simulink model "can8auto"  (R2018a)
settings: Solver=VariableStepAuto  StartTime=0.0  StopTime=5000  RelTol=1e-3
libraries: commcrc2 x20, simulink x20, simulink_extras x5, dspswit3 x5
(part 3 of 7)

== system can8auto/PDO NODO CAN /CAN NODE/NMT Frame generator/11-bit Adder ==
  In1 : Inport
  In2 : Inport  Port=2
  11-bit Adder : Subsystem
  Data Type Conversion : DataTypeConversion
  Demux : Demux  Outputs=11
  Demux1 : Demux  Outputs=11
  Mux : Mux  Inputs=11
  Out1 : Outport
  wires:
  Data Type Conversion/1 -> Out1/1
  Demux1/11 -> 11-bit Adder/22(22)
  Demux1/10 -> 11-bit Adder/21(21)
  Demux1/9 -> 11-bit Adder/20(20)
  Demux1/8 -> 11-bit Adder/19(19)
  Demux1/7 -> 11-bit Adder/18(18)
  Demux1/6 -> 11-bit Adder/17(17)
  Demux1/5 -> 11-bit Adder/16(16)
  Demux1/4 -> 11-bit Adder/15(15)
  Demux1/3 -> 11-bit Adder/14(14)
  Demux1/2 -> 11-bit Adder/13(13)
  Demux1/1 -> 11-bit Adder/12(12)
  Demux/11 -> 11-bit Adder/11(11)
  Demux/10 -> 11-bit Adder/10(10)
  Demux/9 -> 11-bit Adder/9(9)
  Demux/8 -> 11-bit Adder/8(8)
  Demux/7 -> 11-bit Adder/7(7)
  Demux/6 -> 11-bit Adder/6(6)
  Demux/5 -> 11-bit Adder/5(5)
  Demux/4 -> 11-bit Adder/4(4)
  Demux/3 -> 11-bit Adder/3(3)
  Demux/2 -> 11-bit Adder/2(2)
  Demux/1 -> 11-bit Adder/1(1)
  11-bit Adder/11(out11) -> Mux/11
  11-bit Adder/10(out10) -> Mux/10
  11-bit Adder/9(out9) -> Mux/9
  11-bit Adder/8(out8) -> Mux/8
  11-bit Adder/7(out7) -> Mux/7
  11-bit Adder/6(out6) -> Mux/6
  11-bit Adder/5(out5) -> Mux/5
  11-bit Adder/4(out4) -> Mux/4
  11-bit Adder/3(out3) -> Mux/3
  11-bit Adder/2(out2) -> Mux/2
  11-bit Adder/1(out1) -> Mux/1
  In2/1 -> Demux1/1
  In1/1 -> Demux/1
  Mux/1 -> Data Type Conversion/1

== system can8auto/PDO NODO CAN /CAN NODE/NMT Frame generator/BitStuffing ==
  In1 : Inport
  MATLAB Function : MATLAB Function  TreatAsAtomicUnit=on
  Out1 : Outport
  wires:
  In1/1 -> MATLAB Function/1(u)
  MATLAB Function/1(b) -> Out1/1

== system can8auto/PDO NODO CAN /CAN NODE/PDO Frame Generator/Subsystem ==
  Random Bits : Inport
  Length of Field : Inport  Port=2
  1B : Subsystem  TreatAsAtomicUnit=on
  1B1 : Subsystem  TreatAsAtomicUnit=on
  1B2 : Subsystem  TreatAsAtomicUnit=on
  1B3 : Subsystem  TreatAsAtomicUnit=on
  1B4 : Subsystem  TreatAsAtomicUnit=on
  1B5 : Subsystem  TreatAsAtomicUnit=on
  1B6 : Subsystem  TreatAsAtomicUnit=on
  1B7 : Subsystem  TreatAsAtomicUnit=on
  Demux : Demux  Outputs=8
  Index Vector : MultiPortSwitch  Inputs=8  AllowDiffInputSizes=on
  Switch Case : SwitchCase  CaseConditions={1,2,3,4,5,6,7}
  Generated Field : Outport
  wires:
  Switch Case/8 -> 1B7/Action
  1B/1(Out1) -> Index Vector/2
  Demux/3 -> 1B2/3(In3), 1B6/3(In3), 1B4/3(In3), 1B3/3(In3), 1B7/3(In3), 1B5/3(In3)
  Random Bits/1 -> Demux/1
  Switch Case/3 -> 1B2/Action
  Switch Case/6 -> 1B5/Action
  Demux/2 -> 1B2/2(In2), 1B3/2(In2), 1B4/2(In2), 1B5/2(In2), 1B7/2(In2), 1B6/2(In2), 1B1/2(In2)
  1B2/1(Out1) -> Index Vector/4
  Switch Case/5 -> 1B4/Action
  1B3/1(Out1) -> Index Vector/5
  Demux/1 -> 1B1/1(In1), 1B/1(In1), 1B2/1(In1), 1B3/1(In1), 1B4/1(In1), 1B5/1(In1), 1B6/1(In1), 1B7/1(In1)
  Switch Case/2 -> 1B1/Action
  Switch Case/7 -> 1B6/Action
  Demux/4 -> 1B6/4(In4), 1B3/4(In4), 1B7/4(In4), 1B4/4(In4), 1B5/4(In4)
  1B1/1(Out1) -> Index Vector/3
  1B4/1(Out1) -> Index Vector/6
  Demux/8 -> 1B7/8(In8)
  Demux/7 -> 1B6/7(In7), 1B7/7(In7)
  Length of Field/1 -> Switch Case/1, Index Vector/1
  Switch Case/4 -> 1B3/Action
  Demux/5 -> 1B4/5(In5), 1B7/5(In5), 1B6/5(In5), 1B5/5(In5)
  Demux/6 -> 1B5/6(In6), 1B6/6(In6), 1B7/6(In6)
  1B6/1(Out1) -> Index Vector/8
  Switch Case/1 -> 1B/Action
  1B7/1(Out1) -> Index Vector/9
  1B5/1(Out1) -> Index Vector/7
  Index Vector/1 -> Generated Field/1

== system can8auto/PDO NODO CAN /CAN NODE/PDO Frame Generator/Switch Case Action Subsystem ==
  In1 : Inport
  Action Port : ActionPort  ActionType=case
  Out1 : Outport
  wires:
  In1/1 -> Out1/1

== system can8auto/PDO NODO CAN /CAN NODE/PDO Frame Generator/Switch Case Action Subsystem1 ==
  In1 : Inport
  Action Port : ActionPort  ActionType=case
  Out1 : Outport
  wires:
  In1/1 -> Out1/1

== system can8auto/PDO NODO CAN /CAN NODE/PDO Frame Generator/Switch Case Action Subsystem2 ==
  In1 : Inport
  Action Port : ActionPort  ActionType=default
  Out1 : Outport
  wires:
  In1/1 -> Out1/1

== system can8auto/PDO NODO CAN /CAN NODE/SDO Frame generator/BitStuffing ==
  In1 : Inport
  MATLAB Function : MATLAB Function  TreatAsAtomicUnit=on
  Out1 : Outport
  wires:
  In1/1 -> MATLAB Function/1(u)
  MATLAB Function/1(b) -> Out1/1

== system can8auto/PDO NODO CAN /CAN NODE/SDO Frame generator/MUX ==
  Mode : Inport
  Read Client Data : Inport  Port=2
  Write Client Data : Inport  Port=3
  Read Server Data : Inport  Port=4
  Write Server Data : Inport  Port=5
  Complex to Real-Imag : ComplexToRealImag  Output=Real
  MATLAB Function : MATLAB Function  TreatAsAtomicUnit=on
  Vector Concatenate5 : Concatenate  NumInputs=4
  Data to Frame : Outport
  wires:
  Read Server Data/1 -> Vector Concatenate5/3
  Complex to Real-Imag/1 -> Data to Frame/1
  MATLAB Function/1(result) -> Complex to Real-Imag/1
  Read Client Data/1 -> Vector Concatenate5/1
  Vector Concatenate5/1 -> MATLAB Function/2(u1)
  Write Server Data/1 -> Vector Concatenate5/4
  Mode/1 -> MATLAB Function/1(index)
  Write Client Data/1 -> Vector Concatenate5/2

== system can8auto/PDO NODO CAN /CAN NODE/SDO Frame generator/Subsystem ==
  Random Bits : Inport
  Length of Field : Inport  Port=2
  1B : Subsystem  TreatAsAtomicUnit=on
  1B1 : Subsystem  TreatAsAtomicUnit=on
  1B2 : Subsystem  TreatAsAtomicUnit=on
  1B3 : Subsystem  TreatAsAtomicUnit=on
  1B4 : Subsystem  TreatAsAtomicUnit=on
  1B5 : Subsystem  TreatAsAtomicUnit=on
  1B6 : Subsystem  TreatAsAtomicUnit=on
  1B7 : Subsystem  TreatAsAtomicUnit=on
  Demux : Demux  Outputs=8
  Index Vector : MultiPortSwitch  Inputs=8  AllowDiffInputSizes=on
  Switch Case : SwitchCase  CaseConditions={1,2,3,4,5,6,7}
  Generated Field : Outport
  wires:
  Switch Case/8 -> 1B7/Action
  1B/1(Out1) -> Index Vector/2
  Demux/3 -> 1B2/3(In3), 1B6/3(In3), 1B4/3(In3), 1B3/3(In3), 1B7/3(In3), 1B5/3(In3)
  Random Bits/1 -> Demux/1
  Switch Case/3 -> 1B2/Action
  Switch Case/6 -> 1B5/Action
  Demux/2 -> 1B2/2(In2), 1B3/2(In2), 1B4/2(In2), 1B5/2(In2), 1B7/2(In2), 1B6/2(In2), 1B1/2(In2)
  1B2/1(Out1) -> Index Vector/4
  Switch Case/5 -> 1B4/Action
  1B3/1(Out1) -> Index Vector/5
  Demux/1 -> 1B1/1(In1), 1B/1(In1), 1B2/1(In1), 1B3/1(In1), 1B4/1(In1), 1B5/1(In1), 1B6/1(In1), 1B7/1(In1)
  Switch Case/2 -> 1B1/Action
  Switch Case/7 -> 1B6/Action
  Demux/4 -> 1B6/4(In4), 1B3/4(In4), 1B7/4(In4), 1B4/4(In4), 1B5/4(In4)
  1B1/1(Out1) -> Index Vector/3
  1B4/1(Out1) -> Index Vector/6
  Demux/8 -> 1B7/8(In8)
  Demux/7 -> 1B6/7(In7), 1B7/7(In7)
  Length of Field/1 -> Switch Case/1, Index Vector/1
  Switch Case/4 -> 1B3/Action
  Demux/5 -> 1B4/5(In5), 1B7/5(In5), 1B6/5(In5), 1B5/5(In5)
  Demux/6 -> 1B5/6(In6), 1B6/6(In6), 1B7/6(In6)
  1B6/1(Out1) -> Index Vector/8
  Switch Case/1 -> 1B/Action
  1B7/1(Out1) -> Index Vector/9
  1B5/1(Out1) -> Index Vector/7
  Index Vector/1 -> Generated Field/1

== system can8auto/PDO NODO CAN /CAN NODE/SDO Frame generator/Subsystem1 ==
  Random Bits : Inport
  Length of Field : Inport  Port=2
  1B : Subsystem  TreatAsAtomicUnit=on
  1B1 : Subsystem  TreatAsAtomicUnit=on
  1B2 : Subsystem  TreatAsAtomicUnit=on
  1B3 : Subsystem  TreatAsAtomicUnit=on
  1B4 : Subsystem  TreatAsAtomicUnit=on
  1B5 : Subsystem  TreatAsAtomicUnit=on
  1B6 : Subsystem  TreatAsAtomicUnit=on
  1B7 : Subsystem  TreatAsAtomicUnit=on
  Demux : Demux  Outputs=8
  Index Vector : MultiPortSwitch  Inputs=8  AllowDiffInputSizes=on
  Switch Case : SwitchCase  CaseConditions={1,2,3,4,5,6,7}
  Generated Field : Outport
  wires:
  Switch Case/8 -> 1B7/Action
  1B/1(Out1) -> Index Vector/2
  Demux/3 -> 1B2/3(In3), 1B6/3(In3), 1B4/3(In3), 1B3/3(In3), 1B7/3(In3), 1B5/3(In3)
  Random Bits/1 -> Demux/1
  Switch Case/3 -> 1B2/Action
  Switch Case/6 -> 1B5/Action
  Demux/2 -> 1B2/2(In2), 1B3/2(In2), 1B4/2(In2), 1B5/2(In2), 1B7/2(In2), 1B6/2(In2), 1B1/2(In2)
  1B2/1(Out1) -> Index Vector/4
  Switch Case/5 -> 1B4/Action
  1B3/1(Out1) -> Index Vector/5
  Demux/1 -> 1B1/1(In1), 1B/1(In1), 1B2/1(In1), 1B3/1(In1), 1B4/1(In1), 1B5/1(In1), 1B6/1(In1), 1B7/1(In1)
  Switch Case/2 -> 1B1/Action
  Switch Case/7 -> 1B6/Action
  Demux/4 -> 1B6/4(In4), 1B3/4(In4), 1B7/4(In4), 1B4/4(In4), 1B5/4(In4)
  1B1/1(Out1) -> Index Vector/3
  1B4/1(Out1) -> Index Vector/6
  Demux/8 -> 1B7/8(In8)
  Demux/7 -> 1B6/7(In7), 1B7/7(In7)
  Length of Field/1 -> Index Vector/1, Switch Case/1
  Switch Case/4 -> 1B3/Action
  Demux/5 -> 1B4/5(In5), 1B7/5(In5), 1B6/5(In5), 1B5/5(In5)
  Demux/6 -> 1B5/6(In6), 1B6/6(In6), 1B7/6(In6)
  1B6/1(Out1) -> Index Vector/8
  Switch Case/1 -> 1B/Action
  1B7/1(Out1) -> Index Vector/9
  1B5/1(Out1) -> Index Vector/7
  Index Vector/1 -> Generated Field/1

== system can8auto/PDO NODO CAN /CAN NODE/SDO Frame generator/Subsystem2 ==
  Random Bits : Inport
  Length of Field : Inport  Port=2
  1B : Subsystem  TreatAsAtomicUnit=on
  1B1 : Subsystem  TreatAsAtomicUnit=on
  1B2 : Subsystem  TreatAsAtomicUnit=on
  1B3 : Subsystem  TreatAsAtomicUnit=on
  1B4 : Subsystem  TreatAsAtomicUnit=on
  1B5 : Subsystem  TreatAsAtomicUnit=on
  1B6 : Subsystem  TreatAsAtomicUnit=on
  1B7 : Subsystem  TreatAsAtomicUnit=on
  Demux : Demux  Outputs=8
  Index Vector : MultiPortSwitch  Inputs=8  AllowDiffInputSizes=on
  Switch Case : SwitchCase  CaseConditions={1,2,3,4,5,6,7}
  Generated Field : Outport
  wires:
  Switch Case/8 -> 1B7/Action
  1B/1(Out1) -> Index Vector/2
  Demux/3 -> 1B2/3(In3), 1B6/3(In3), 1B4/3(In3), 1B3/3(In3), 1B7/3(In3), 1B5/3(In3)
  Random Bits/1 -> Demux/1
  Switch Case/3 -> 1B2/Action
  Switch Case/6 -> 1B5/Action
  Demux/2 -> 1B2/2(In2), 1B3/2(In2), 1B4/2(In2), 1B5/2(In2), 1B7/2(In2), 1B6/2(In2), 1B1/2(In2)
  1B2/1(Out1) -> Index Vector/4
  Switch Case/5 -> 1B4/Action
  1B3/1(Out1) -> Index Vector/5
  Demux/1 -> 1B1/1(In1), 1B/1(In1), 1B2/1(In1), 1B3/1(In1), 1B4/1(In1), 1B5/1(In1), 1B6/1(In1), 1B7/1(In1)
  Switch Case/2 -> 1B1/Action
  Switch Case/7 -> 1B6/Action
  Demux/4 -> 1B6/4(In4), 1B3/4(In4), 1B7/4(In4), 1B4/4(In4), 1B5/4(In4)
  1B1/1(Out1) -> Index Vector/3
  1B4/1(Out1) -> Index Vector/6
  Demux/8 -> 1B7/8(In8)
  Demux/7 -> 1B6/7(In7), 1B7/7(In7)
  Length of Field/1 -> Switch Case/1, Index Vector/1
  Switch Case/4 -> 1B3/Action
  Demux/5 -> 1B4/5(In5), 1B7/5(In5), 1B6/5(In5), 1B5/5(In5)
  Demux/6 -> 1B5/6(In6), 1B6/6(In6), 1B7/6(In6)
  1B6/1(Out1) -> Index Vector/8
  Switch Case/1 -> 1B/Action
  1B7/1(Out1) -> Index Vector/9
  1B5/1(Out1) -> Index Vector/7
  Index Vector/1 -> Generated Field/1

== system can8auto/PDO NODO CAN /CAN NODE/SDO Frame generator/Subsystem3 ==
  Random Bits : Inport
  Length of Field : Inport  Port=2
  1B : Subsystem  TreatAsAtomicUnit=on
  1B1 : Subsystem  TreatAsAtomicUnit=on
  1B2 : Subsystem  TreatAsAtomicUnit=on
  1B3 : Subsystem  TreatAsAtomicUnit=on
  1B4 : Subsystem  TreatAsAtomicUnit=on
  1B5 : Subsystem  TreatAsAtomicUnit=on
  1B6 : Subsystem  TreatAsAtomicUnit=on
  1B7 : Subsystem  TreatAsAtomicUnit=on
  Demux : Demux  Outputs=8
  Index Vector : MultiPortSwitch  Inputs=8  AllowDiffInputSizes=on
  Switch Case : SwitchCase  CaseConditions={1,2,3,4,5,6,7}
  Generated Field : Outport
  wires:
  Switch Case/8 -> 1B7/Action
  1B/1(Out1) -> Index Vector/2
  Demux/3 -> 1B2/3(In3), 1B6/3(In3), 1B4/3(In3), 1B3/3(In3), 1B7/3(In3), 1B5/3(In3)
  Random Bits/1 -> Demux/1
  Switch Case/3 -> 1B2/Action
  Switch Case/6 -> 1B5/Action
  Demux/2 -> 1B2/2(In2), 1B3/2(In2), 1B4/2(In2), 1B5/2(In2), 1B7/2(In2), 1B6/2(In2), 1B1/2(In2)
  1B2/1(Out1) -> Index Vector/4
  Switch Case/5 -> 1B4/Action
  1B3/1(Out1) -> Index Vector/5
  Demux/1 -> 1B1/1(In1), 1B/1(In1), 1B2/1(In1), 1B3/1(In1), 1B4/1(In1), 1B5/1(In1), 1B6/1(In1), 1B7/1(In1)
  Switch Case/2 -> 1B1/Action
  Switch Case/7 -> 1B6/Action
  Demux/4 -> 1B6/4(In4), 1B3/4(In4), 1B7/4(In4), 1B4/4(In4), 1B5/4(In4)
  1B1/1(Out1) -> Index Vector/3
  1B4/1(Out1) -> Index Vector/6
  Demux/8 -> 1B7/8(In8)
  Demux/7 -> 1B6/7(In7), 1B7/7(In7)
  Length of Field/1 -> Switch Case/1, Index Vector/1
  Switch Case/4 -> 1B3/Action
  Demux/5 -> 1B4/5(In5), 1B7/5(In5), 1B6/5(In5), 1B5/5(In5)
  Demux/6 -> 1B5/6(In6), 1B6/6(In6), 1B7/6(In6)
  1B6/1(Out1) -> Index Vector/8
  Switch Case/1 -> 1B/Action
  1B7/1(Out1) -> Index Vector/9
  1B5/1(Out1) -> Index Vector/7
  Index Vector/1 -> Generated Field/1

== system can8auto/PDO NODO CAN /CAN NODE/SYNC Frame Generator/BitStuffing ==
  In1 : Inport
  MATLAB Function : MATLAB Function  TreatAsAtomicUnit=on
  Out1 : Outport
  wires:
  In1/1 -> MATLAB Function/1(u)
  MATLAB Function/1(b) -> Out1/1

== system can8auto/SDO NODO CAN/CAN NODE/Bootup Frame generator/11-bit Adder ==
  In1 : Inport
  In2 : Inport  Port=2
  8-bit Adder : Subsystem
  Data Type Conversion : DataTypeConversion
  Demux : Demux  Outputs=11
  Demux1 : Demux  Outputs=11
  Mux : Mux  Inputs=11
  Out1 : Outport
  wires:
  Data Type Conversion/1 -> Out1/1
  Mux/1 -> Data Type Conversion/1
  Demux1/11 -> 8-bit Adder/22(22)
  Demux1/10 -> 8-bit Adder/21(21)
  Demux1/9 -> 8-bit Adder/20(20)
  Demux1/8 -> 8-bit Adder/19(19)
  Demux1/7 -> 8-bit Adder/18(18)
  Demux1/6 -> 8-bit Adder/17(17)
  Demux1/5 -> 8-bit Adder/16(16)
  Demux1/4 -> 8-bit Adder/15(15)
  Demux1/3 -> 8-bit Adder/14(14)
  Demux1/2 -> 8-bit Adder/13(13)
  Demux1/1 -> 8-bit Adder/12(12)
  Demux/11 -> 8-bit Adder/11(11)
  Demux/10 -> 8-bit Adder/10(10)
  Demux/9 -> 8-bit Adder/9(9)
  Demux/8 -> 8-bit Adder/8(8)
  Demux/7 -> 8-bit Adder/7(7)
  Demux/6 -> 8-bit Adder/6(6)
  Demux/5 -> 8-bit Adder/5(5)
  Demux/4 -> 8-bit Adder/4(4)
  Demux/3 -> 8-bit Adder/3(3)
  Demux/2 -> 8-bit Adder/2(2)
  Demux/1 -> 8-bit Adder/1(1)
  8-bit Adder/11(out11) -> Mux/11
  8-bit Adder/10(out10) -> Mux/10
  8-bit Adder/9(out9) -> Mux/9
  8-bit Adder/8(out8) -> Mux/8
  8-bit Adder/7(out7) -> Mux/7
  8-bit Adder/6(out6) -> Mux/6
  8-bit Adder/5(out5) -> Mux/5
  8-bit Adder/4(out4) -> Mux/4
  8-bit Adder/3(out3) -> Mux/3
  8-bit Adder/2(out2) -> Mux/2
  8-bit Adder/1(out1) -> Mux/1
  In2/1 -> Demux1/1
  In1/1 -> Demux/1

== system can8auto/SDO NODO CAN/CAN NODE/Bootup Frame generator/BitStuffing ==
  In1 : Inport
  MATLAB Function : MATLAB Function  TreatAsAtomicUnit=on
  Out1 : Outport
  wires:
  In1/1 -> MATLAB Function/1(u)
  MATLAB Function/1(b) -> Out1/1

== system can8auto/SDO NODO CAN/CAN NODE/NMT Frame generator/11-bit Adder ==
  In1 : Inport
  In2 : Inport  Port=2
  11-bit Adder : Subsystem
  Data Type Conversion : DataTypeConversion
  Demux : Demux  Outputs=11
  Demux1 : Demux  Outputs=11
  Mux : Mux  Inputs=11
  Out1 : Outport
  wires:
  Data Type Conversion/1 -> Out1/1
  Demux1/11 -> 11-bit Adder/22(22)
  Demux1/10 -> 11-bit Adder/21(21)
  Demux1/9 -> 11-bit Adder/20(20)
  Demux1/8 -> 11-bit Adder/19(19)
  Demux1/7 -> 11-bit Adder/18(18)
  Demux1/6 -> 11-bit Adder/17(17)
  Demux1/5 -> 11-bit Adder/16(16)
  Demux1/4 -> 11-bit Adder/15(15)
  Demux1/3 -> 11-bit Adder/14(14)
  Demux1/2 -> 11-bit Adder/13(13)
  Demux1/1 -> 11-bit Adder/12(12)
  Demux/11 -> 11-bit Adder/11(11)
  Demux/10 -> 11-bit Adder/10(10)
  Demux/9 -> 11-bit Adder/9(9)
  Demux/8 -> 11-bit Adder/8(8)
  Demux/7 -> 11-bit Adder/7(7)
  Demux/6 -> 11-bit Adder/6(6)
  Demux/5 -> 11-bit Adder/5(5)
  Demux/4 -> 11-bit Adder/4(4)
  Demux/3 -> 11-bit Adder/3(3)
  Demux/2 -> 11-bit Adder/2(2)
  Demux/1 -> 11-bit Adder/1(1)
  11-bit Adder/11(out11) -> Mux/11
  11-bit Adder/10(out10) -> Mux/10
  11-bit Adder/9(out9) -> Mux/9
  11-bit Adder/8(out8) -> Mux/8
  11-bit Adder/7(out7) -> Mux/7
  11-bit Adder/6(out6) -> Mux/6
  11-bit Adder/5(out5) -> Mux/5
  11-bit Adder/4(out4) -> Mux/4
  11-bit Adder/3(out3) -> Mux/3
  11-bit Adder/2(out2) -> Mux/2
  11-bit Adder/1(out1) -> Mux/1
  In2/1 -> Demux1/1
  In1/1 -> Demux/1
  Mux/1 -> Data Type Conversion/1

== system can8auto/SDO NODO CAN/CAN NODE/NMT Frame generator/BitStuffing ==
  In1 : Inport
  MATLAB Function : MATLAB Function  TreatAsAtomicUnit=on
  Out1 : Outport
  wires:
  In1/1 -> MATLAB Function/1(u)
  MATLAB Function/1(b) -> Out1/1

== system can8auto/SDO NODO CAN/CAN NODE/PDO Frame Generator/Subsystem ==
  Random Bits : Inport
  Length of Field : Inport  Port=2
  1B : Subsystem  TreatAsAtomicUnit=on
  1B1 : Subsystem  TreatAsAtomicUnit=on
  1B2 : Subsystem  TreatAsAtomicUnit=on
  1B3 : Subsystem  TreatAsAtomicUnit=on
  1B4 : Subsystem  TreatAsAtomicUnit=on
  1B5 : Subsystem  TreatAsAtomicUnit=on
  1B6 : Subsystem  TreatAsAtomicUnit=on
  1B7 : Subsystem  TreatAsAtomicUnit=on
  Demux : Demux  Outputs=8
  Index Vector : MultiPortSwitch  Inputs=8  AllowDiffInputSizes=on
  Switch Case : SwitchCase  CaseConditions={1,2,3,4,5,6,7}
  Generated Field : Outport
  wires:
  Switch Case/8 -> 1B7/Action
  1B/1(Out1) -> Index Vector/2
  Demux/3 -> 1B2/3(In3), 1B6/3(In3), 1B4/3(In3), 1B3/3(In3), 1B7/3(In3), 1B5/3(In3)
  Random Bits/1 -> Demux/1
  Switch Case/3 -> 1B2/Action
  Switch Case/6 -> 1B5/Action
  Demux/2 -> 1B2/2(In2), 1B3/2(In2), 1B4/2(In2), 1B5/2(In2), 1B7/2(In2), 1B6/2(In2), 1B1/2(In2)
  1B2/1(Out1) -> Index Vector/4
  Switch Case/5 -> 1B4/Action
  1B3/1(Out1) -> Index Vector/5
  Demux/1 -> 1B1/1(In1), 1B/1(In1), 1B2/1(In1), 1B3/1(In1), 1B4/1(In1), 1B5/1(In1), 1B6/1(In1), 1B7/1(In1)
  Switch Case/2 -> 1B1/Action
  Switch Case/7 -> 1B6/Action
  Demux/4 -> 1B6/4(In4), 1B3/4(In4), 1B7/4(In4), 1B4/4(In4), 1B5/4(In4)
  1B1/1(Out1) -> Index Vector/3
  1B4/1(Out1) -> Index Vector/6
  Demux/8 -> 1B7/8(In8)
  Demux/7 -> 1B6/7(In7), 1B7/7(In7)
  Length of Field/1 -> Switch Case/1, Index Vector/1
  Switch Case/4 -> 1B3/Action
  Demux/5 -> 1B4/5(In5), 1B7/5(In5), 1B6/5(In5), 1B5/5(In5)
  Demux/6 -> 1B5/6(In6), 1B6/6(In6), 1B7/6(In6)
  1B6/1(Out1) -> Index Vector/8
  Switch Case/1 -> 1B/Action
  1B7/1(Out1) -> Index Vector/9
  1B5/1(Out1) -> Index Vector/7
  Index Vector/1 -> Generated Field/1

== system can8auto/SDO NODO CAN/CAN NODE/PDO Frame Generator/Switch Case Action Subsystem ==
  In1 : Inport
  Action Port : ActionPort  ActionType=case
  Out1 : Outport
  wires:
  In1/1 -> Out1/1

== system can8auto/SDO NODO CAN/CAN NODE/PDO Frame Generator/Switch Case Action Subsystem1 ==
  In1 : Inport
  Action Port : ActionPort  ActionType=case
  Out1 : Outport
  wires:
  In1/1 -> Out1/1

== system can8auto/SDO NODO CAN/CAN NODE/PDO Frame Generator/Switch Case Action Subsystem2 ==
  In1 : Inport
  Action Port : ActionPort  ActionType=default
  Out1 : Outport
  wires:
  In1/1 -> Out1/1

== system can8auto/SDO NODO CAN/CAN NODE/SDO Frame generator/BitStuffing ==
  In1 : Inport
  MATLAB Function : MATLAB Function  TreatAsAtomicUnit=on
  Out1 : Outport
  wires:
  In1/1 -> MATLAB Function/1(u)
  MATLAB Function/1(b) -> Out1/1

== system can8auto/SDO NODO CAN/CAN NODE/SDO Frame generator/MUX ==
  Mode : Inport
  Read Client Data : Inport  Port=2
  Write Client Data : Inport  Port=3
  Read Server Data : Inport  Port=4
  Write Server Data : Inport  Port=5
  Complex to Real-Imag : ComplexToRealImag  Output=Real
  MATLAB Function : MATLAB Function  TreatAsAtomicUnit=on
  Vector Concatenate5 : Concatenate  NumInputs=4
  Data to Frame : Outport
  wires:
  Read Server Data/1 -> Vector Concatenate5/3
  Complex to Real-Imag/1 -> Data to Frame/1
  MATLAB Function/1(result) -> Complex to Real-Imag/1
  Read Client Data/1 -> Vector Concatenate5/1
  Vector Concatenate5/1 -> MATLAB Function/2(u1)
  Write Server Data/1 -> Vector Concatenate5/4
  Mode/1 -> MATLAB Function/1(index)
  Write Client Data/1 -> Vector Concatenate5/2

== system can8auto/SDO NODO CAN/CAN NODE/SDO Frame generator/Subsystem ==
  Random Bits : Inport
  Length of Field : Inport  Port=2
  1B : Subsystem  TreatAsAtomicUnit=on
  1B1 : Subsystem  TreatAsAtomicUnit=on
  1B2 : Subsystem  TreatAsAtomicUnit=on
  1B3 : Subsystem  TreatAsAtomicUnit=on
  1B4 : Subsystem  TreatAsAtomicUnit=on
  1B5 : Subsystem  TreatAsAtomicUnit=on
  1B6 : Subsystem  TreatAsAtomicUnit=on
  1B7 : Subsystem  TreatAsAtomicUnit=on
  Demux : Demux  Outputs=8
  Index Vector : MultiPortSwitch  Inputs=8  AllowDiffInputSizes=on
  Switch Case : SwitchCase  CaseConditions={1,2,3,4,5,6,7}
  Generated Field : Outport
  wires:
  Switch Case/8 -> 1B7/Action
  1B/1(Out1) -> Index Vector/2
  Demux/3 -> 1B2/3(In3), 1B6/3(In3), 1B4/3(In3), 1B3/3(In3), 1B7/3(In3), 1B5/3(In3)
  Random Bits/1 -> Demux/1
  Switch Case/3 -> 1B2/Action
  Switch Case/6 -> 1B5/Action
  Demux/2 -> 1B2/2(In2), 1B3/2(In2), 1B4/2(In2), 1B5/2(In2), 1B7/2(In2), 1B6/2(In2), 1B1/2(In2)
  1B2/1(Out1) -> Index Vector/4
  Switch Case/5 -> 1B4/Action
  1B3/1(Out1) -> Index Vector/5
  Demux/1 -> 1B1/1(In1), 1B/1(In1), 1B2/1(In1), 1B3/1(In1), 1B4/1(In1), 1B5/1(In1), 1B6/1(In1), 1B7/1(In1)
  Switch Case/2 -> 1B1/Action
  Switch Case/7 -> 1B6/Action
  Demux/4 -> 1B6/4(In4), 1B3/4(In4), 1B7/4(In4), 1B4/4(In4), 1B5/4(In4)
  1B1/1(Out1) -> Index Vector/3
  1B4/1(Out1) -> Index Vector/6
  Demux/8 -> 1B7/8(In8)
  Demux/7 -> 1B6/7(In7), 1B7/7(In7)
  Length of Field/1 -> Switch Case/1, Index Vector/1
  Switch Case/4 -> 1B3/Action
  Demux/5 -> 1B4/5(In5), 1B7/5(In5), 1B6/5(In5), 1B5/5(In5)
  Demux/6 -> 1B5/6(In6), 1B6/6(In6), 1B7/6(In6)
  1B6/1(Out1) -> Index Vector/8
  Switch Case/1 -> 1B/Action
  1B7/1(Out1) -> Index Vector/9
  1B5/1(Out1) -> Index Vector/7
  Index Vector/1 -> Generated Field/1

== system can8auto/SDO NODO CAN/CAN NODE/SDO Frame generator/Subsystem1 ==
  Random Bits : Inport
  Length of Field : Inport  Port=2
  1B : Subsystem  TreatAsAtomicUnit=on
  1B1 : Subsystem  TreatAsAtomicUnit=on
  1B2 : Subsystem  TreatAsAtomicUnit=on
  1B3 : Subsystem  TreatAsAtomicUnit=on
  1B4 : Subsystem  TreatAsAtomicUnit=on
  1B5 : Subsystem  TreatAsAtomicUnit=on
  1B6 : Subsystem  TreatAsAtomicUnit=on
  1B7 : Subsystem  TreatAsAtomicUnit=on
  Demux : Demux  Outputs=8
  Index Vector : MultiPortSwitch  Inputs=8  AllowDiffInputSizes=on
  Switch Case : SwitchCase  CaseConditions={1,2,3,4,5,6,7}
  Generated Field : Outport
  wires:
  Switch Case/8 -> 1B7/Action
  1B/1(Out1) -> Index Vector/2
  Demux/3 -> 1B2/3(In3), 1B6/3(In3), 1B4/3(In3), 1B3/3(In3), 1B7/3(In3), 1B5/3(In3)
  Random Bits/1 -> Demux/1
  Switch Case/3 -> 1B2/Action
  Switch Case/6 -> 1B5/Action
  Demux/2 -> 1B2/2(In2), 1B3/2(In2), 1B4/2(In2), 1B5/2(In2), 1B7/2(In2), 1B6/2(In2), 1B1/2(In2)
  1B2/1(Out1) -> Index Vector/4
  Switch Case/5 -> 1B4/Action
  1B3/1(Out1) -> Index Vector/5
  Demux/1 -> 1B1/1(In1), 1B/1(In1), 1B2/1(In1), 1B3/1(In1), 1B4/1(In1), 1B5/1(In1), 1B6/1(In1), 1B7/1(In1)
  Switch Case/2 -> 1B1/Action
  Switch Case/7 -> 1B6/Action
  Demux/4 -> 1B6/4(In4), 1B3/4(In4), 1B7/4(In4), 1B4/4(In4), 1B5/4(In4)
  1B1/1(Out1) -> Index Vector/3
  1B4/1(Out1) -> Index Vector/6
  Demux/8 -> 1B7/8(In8)
  Demux/7 -> 1B6/7(In7), 1B7/7(In7)
  Length of Field/1 -> Index Vector/1, Switch Case/1
  Switch Case/4 -> 1B3/Action
  Demux/5 -> 1B4/5(In5), 1B7/5(In5), 1B6/5(In5), 1B5/5(In5)
  Demux/6 -> 1B5/6(In6), 1B6/6(In6), 1B7/6(In6)
  1B6/1(Out1) -> Index Vector/8
  Switch Case/1 -> 1B/Action
  1B7/1(Out1) -> Index Vector/9
  1B5/1(Out1) -> Index Vector/7
  Index Vector/1 -> Generated Field/1

== system can8auto/SDO NODO CAN/CAN NODE/SDO Frame generator/Subsystem2 ==
  Random Bits : Inport
  Length of Field : Inport  Port=2
  1B : Subsystem  TreatAsAtomicUnit=on
  1B1 : Subsystem  TreatAsAtomicUnit=on
  1B2 : Subsystem  TreatAsAtomicUnit=on
  1B3 : Subsystem  TreatAsAtomicUnit=on
  1B4 : Subsystem  TreatAsAtomicUnit=on
  1B5 : Subsystem  TreatAsAtomicUnit=on
  1B6 : Subsystem  TreatAsAtomicUnit=on
  1B7 : Subsystem  TreatAsAtomicUnit=on
  Demux : Demux  Outputs=8
  Index Vector : MultiPortSwitch  Inputs=8  AllowDiffInputSizes=on
  Switch Case : SwitchCase  CaseConditions={1,2,3,4,5,6,7}
  Generated Field : Outport
  wires:
  Switch Case/8 -> 1B7/Action
  1B/1(Out1) -> Index Vector/2
  Demux/3 -> 1B2/3(In3), 1B6/3(In3), 1B4/3(In3), 1B3/3(In3), 1B7/3(In3), 1B5/3(In3)
  Random Bits/1 -> Demux/1
  Switch Case/3 -> 1B2/Action
  Switch Case/6 -> 1B5/Action
  Demux/2 -> 1B2/2(In2), 1B3/2(In2), 1B4/2(In2), 1B5/2(In2), 1B7/2(In2), 1B6/2(In2), 1B1/2(In2)
  1B2/1(Out1) -> Index Vector/4
  Switch Case/5 -> 1B4/Action
  1B3/1(Out1) -> Index Vector/5
  Demux/1 -> 1B1/1(In1), 1B/1(In1), 1B2/1(In1), 1B3/1(In1), 1B4/1(In1), 1B5/1(In1), 1B6/1(In1), 1B7/1(In1)
  Switch Case/2 -> 1B1/Action
  Switch Case/7 -> 1B6/Action
  Demux/4 -> 1B6/4(In4), 1B3/4(In4), 1B7/4(In4), 1B4/4(In4), 1B5/4(In4)
  1B1/1(Out1) -> Index Vector/3
  1B4/1(Out1) -> Index Vector/6
  Demux/8 -> 1B7/8(In8)
  Demux/7 -> 1B6/7(In7), 1B7/7(In7)
  Length of Field/1 -> Switch Case/1, Index Vector/1
  Switch Case/4 -> 1B3/Action
  Demux/5 -> 1B4/5(In5), 1B7/5(In5), 1B6/5(In5), 1B5/5(In5)
  Demux/6 -> 1B5/6(In6), 1B6/6(In6), 1B7/6(In6)
  1B6/1(Out1) -> Index Vector/8
  Switch Case/1 -> 1B/Action
  1B7/1(Out1) -> Index Vector/9
  1B5/1(Out1) -> Index Vector/7
  Index Vector/1 -> Generated Field/1

== system can8auto/SDO NODO CAN/CAN NODE/SDO Frame generator/Subsystem3 ==
  Random Bits : Inport
  Length of Field : Inport  Port=2
  1B : Subsystem  TreatAsAtomicUnit=on
  1B1 : Subsystem  TreatAsAtomicUnit=on
  1B2 : Subsystem  TreatAsAtomicUnit=on
  1B3 : Subsystem  TreatAsAtomicUnit=on
  1B4 : Subsystem  TreatAsAtomicUnit=on
  1B5 : Subsystem  TreatAsAtomicUnit=on
  1B6 : Subsystem  TreatAsAtomicUnit=on
  1B7 : Subsystem  TreatAsAtomicUnit=on
  Demux : Demux  Outputs=8
  Index Vector : MultiPortSwitch  Inputs=8  AllowDiffInputSizes=on
  Switch Case : SwitchCase  CaseConditions={1,2,3,4,5,6,7}
  Generated Field : Outport
  wires:
  Switch Case/8 -> 1B7/Action
  1B/1(Out1) -> Index Vector/2
  Demux/3 -> 1B2/3(In3), 1B6/3(In3), 1B4/3(In3), 1B3/3(In3), 1B7/3(In3), 1B5/3(In3)
  Random Bits/1 -> Demux/1
  Switch Case/3 -> 1B2/Action
  Switch Case/6 -> 1B5/Action
  Demux/2 -> 1B2/2(In2), 1B3/2(In2), 1B4/2(In2), 1B5/2(In2), 1B7/2(In2), 1B6/2(In2), 1B1/2(In2)
  1B2/1(Out1) -> Index Vector/4
  Switch Case/5 -> 1B4/Action
  1B3/1(Out1) -> Index Vector/5
  Demux/1 -> 1B1/1(In1), 1B/1(In1), 1B2/1(In1), 1B3/1(In1), 1B4/1(In1), 1B5/1(In1), 1B6/1(In1), 1B7/1(In1)
  Switch Case/2 -> 1B1/Action
  Switch Case/7 -> 1B6/Action
  Demux/4 -> 1B6/4(In4), 1B3/4(In4), 1B7/4(In4), 1B4/4(In4), 1B5/4(In4)
  1B1/1(Out1) -> Index Vector/3
  1B4/1(Out1) -> Index Vector/6
  Demux/8 -> 1B7/8(In8)
  Demux/7 -> 1B6/7(In7), 1B7/7(In7)
  Length of Field/1 -> Switch Case/1, Index Vector/1
  Switch Case/4 -> 1B3/Action
  Demux/5 -> 1B4/5(In5), 1B7/5(In5), 1B6/5(In5), 1B5/5(In5)
  Demux/6 -> 1B5/6(In6), 1B6/6(In6), 1B7/6(In6)
  1B6/1(Out1) -> Index Vector/8
  Switch Case/1 -> 1B/Action
  1B7/1(Out1) -> Index Vector/9
  1B5/1(Out1) -> Index Vector/7
  Index Vector/1 -> Generated Field/1

== system can8auto/SDO NODO CAN/CAN NODE/SYNC Frame Generator/BitStuffing ==
  In1 : Inport
  MATLAB Function : MATLAB Function  TreatAsAtomicUnit=on
  Out1 : Outport
  wires:
  In1/1 -> MATLAB Function/1(u)
  MATLAB Function/1(b) -> Out1/1

== system can8auto/SYNC PRODUCER/CAN NODE/Bootup Frame generator/11-bit Adder ==
  In1 : Inport
  In2 : Inport  Port=2
  8-bit Adder : Subsystem
  Data Type Conversion : DataTypeConversion
  Demux : Demux  Outputs=11
  Demux1 : Demux  Outputs=11
  Mux : Mux  Inputs=11
  Out1 : Outport
  wires:
  Data Type Conversion/1 -> Out1/1
  Mux/1 -> Data Type Conversion/1
  Demux1/11 -> 8-bit Adder/22(22)
  Demux1/10 -> 8-bit Adder/21(21)
  Demux1/9 -> 8-bit Adder/20(20)
  Demux1/8 -> 8-bit Adder/19(19)
  Demux1/7 -> 8-bit Adder/18(18)
  Demux1/6 -> 8-bit Adder/17(17)
  Demux1/5 -> 8-bit Adder/16(16)
  Demux1/4 -> 8-bit Adder/15(15)
  Demux1/3 -> 8-bit Adder/14(14)
  Demux1/2 -> 8-bit Adder/13(13)
  Demux1/1 -> 8-bit Adder/12(12)
  Demux/11 -> 8-bit Adder/11(11)
  Demux/10 -> 8-bit Adder/10(10)
  Demux/9 -> 8-bit Adder/9(9)
  Demux/8 -> 8-bit Adder/8(8)
  Demux/7 -> 8-bit Adder/7(7)
  Demux/6 -> 8-bit Adder/6(6)
  Demux/5 -> 8-bit Adder/5(5)
  Demux/4 -> 8-bit Adder/4(4)
  Demux/3 -> 8-bit Adder/3(3)
  Demux/2 -> 8-bit Adder/2(2)
  Demux/1 -> 8-bit Adder/1(1)
  8-bit Adder/11(out11) -> Mux/11
  8-bit Adder/10(out10) -> Mux/10
  8-bit Adder/9(out9) -> Mux/9
  8-bit Adder/8(out8) -> Mux/8
  8-bit Adder/7(out7) -> Mux/7
  8-bit Adder/6(out6) -> Mux/6
  8-bit Adder/5(out5) -> Mux/5
  8-bit Adder/4(out4) -> Mux/4
  8-bit Adder/3(out3) -> Mux/3
  8-bit Adder/2(out2) -> Mux/2
  8-bit Adder/1(out1) -> Mux/1
  In2/1 -> Demux1/1
  In1/1 -> Demux/1

== system can8auto/SYNC PRODUCER/CAN NODE/Bootup Frame generator/BitStuffing ==
  In1 : Inport
  MATLAB Function : MATLAB Function  TreatAsAtomicUnit=on
  Out1 : Outport
  wires:
  In1/1 -> MATLAB Function/1(u)
  MATLAB Function/1(b) -> Out1/1

== system can8auto/SYNC PRODUCER/CAN NODE/NMT Frame generator/11-bit Adder ==
  In1 : Inport
  In2 : Inport  Port=2
  11-bit Adder : Subsystem
  Data Type Conversion : DataTypeConversion
  Demux : Demux  Outputs=11
  Demux1 : Demux  Outputs=11
  Mux : Mux  Inputs=11
  Out1 : Outport
  wires:
  Data Type Conversion/1 -> Out1/1
  Demux1/11 -> 11-bit Adder/22(22)
  Demux1/10 -> 11-bit Adder/21(21)
  Demux1/9 -> 11-bit Adder/20(20)
  Demux1/8 -> 11-bit Adder/19(19)
  Demux1/7 -> 11-bit Adder/18(18)
  Demux1/6 -> 11-bit Adder/17(17)
  Demux1/5 -> 11-bit Adder/16(16)
  Demux1/4 -> 11-bit Adder/15(15)
  Demux1/3 -> 11-bit Adder/14(14)
  Demux1/2 -> 11-bit Adder/13(13)
  Demux1/1 -> 11-bit Adder/12(12)
  Demux/11 -> 11-bit Adder/11(11)
  Demux/10 -> 11-bit Adder/10(10)
  Demux/9 -> 11-bit Adder/9(9)
  Demux/8 -> 11-bit Adder/8(8)
  Demux/7 -> 11-bit Adder/7(7)
  Demux/6 -> 11-bit Adder/6(6)
  Demux/5 -> 11-bit Adder/5(5)
  Demux/4 -> 11-bit Adder/4(4)
  Demux/3 -> 11-bit Adder/3(3)
  Demux/2 -> 11-bit Adder/2(2)
  Demux/1 -> 11-bit Adder/1(1)
  11-bit Adder/11(out11) -> Mux/11
  11-bit Adder/10(out10) -> Mux/10
  11-bit Adder/9(out9) -> Mux/9
  11-bit Adder/8(out8) -> Mux/8
  11-bit Adder/7(out7) -> Mux/7
  11-bit Adder/6(out6) -> Mux/6
  11-bit Adder/5(out5) -> Mux/5
  11-bit Adder/4(out4) -> Mux/4
  11-bit Adder/3(out3) -> Mux/3
  11-bit Adder/2(out2) -> Mux/2
  11-bit Adder/1(out1) -> Mux/1
  In2/1 -> Demux1/1
  In1/1 -> Demux/1
  Mux/1 -> Data Type Conversion/1

== system can8auto/SYNC PRODUCER/CAN NODE/NMT Frame generator/BitStuffing ==
  In1 : Inport
  MATLAB Function : MATLAB Function  TreatAsAtomicUnit=on
  Out1 : Outport
  wires:
  In1/1 -> MATLAB Function/1(u)
  MATLAB Function/1(b) -> Out1/1

== system can8auto/SYNC PRODUCER/CAN NODE/PDO Frame Generator/Subsystem ==
  Random Bits : Inport
  Length of Field : Inport  Port=2
  1B : Subsystem  TreatAsAtomicUnit=on
  1B1 : Subsystem  TreatAsAtomicUnit=on
  1B2 : Subsystem  TreatAsAtomicUnit=on
  1B3 : Subsystem  TreatAsAtomicUnit=on
  1B4 : Subsystem  TreatAsAtomicUnit=on
  1B5 : Subsystem  TreatAsAtomicUnit=on
  1B6 : Subsystem  TreatAsAtomicUnit=on
  1B7 : Subsystem  TreatAsAtomicUnit=on
  Demux : Demux  Outputs=8
  Index Vector : MultiPortSwitch  Inputs=8  AllowDiffInputSizes=on
  Switch Case : SwitchCase  CaseConditions={1,2,3,4,5,6,7}
  Generated Field : Outport
  wires:
  Switch Case/8 -> 1B7/Action
  1B/1(Out1) -> Index Vector/2
  Demux/3 -> 1B2/3(In3), 1B6/3(In3), 1B4/3(In3), 1B3/3(In3), 1B7/3(In3), 1B5/3(In3)
  Random Bits/1 -> Demux/1
  Switch Case/3 -> 1B2/Action
  Switch Case/6 -> 1B5/Action
  Demux/2 -> 1B2/2(In2), 1B3/2(In2), 1B4/2(In2), 1B5/2(In2), 1B7/2(In2), 1B6/2(In2), 1B1/2(In2)
  1B2/1(Out1) -> Index Vector/4
  Switch Case/5 -> 1B4/Action
  1B3/1(Out1) -> Index Vector/5
  Demux/1 -> 1B1/1(In1), 1B/1(In1), 1B2/1(In1), 1B3/1(In1), 1B4/1(In1), 1B5/1(In1), 1B6/1(In1), 1B7/1(In1)
  Switch Case/2 -> 1B1/Action
  Switch Case/7 -> 1B6/Action
  Demux/4 -> 1B6/4(In4), 1B3/4(In4), 1B7/4(In4), 1B4/4(In4), 1B5/4(In4)
  1B1/1(Out1) -> Index Vector/3
  1B4/1(Out1) -> Index Vector/6
  Demux/8 -> 1B7/8(In8)
  Demux/7 -> 1B6/7(In7), 1B7/7(In7)
  Length of Field/1 -> Switch Case/1, Index Vector/1
  Switch Case/4 -> 1B3/Action
  Demux/5 -> 1B4/5(In5), 1B7/5(In5), 1B6/5(In5), 1B5/5(In5)
  Demux/6 -> 1B5/6(In6), 1B6/6(In6), 1B7/6(In6)
  1B6/1(Out1) -> Index Vector/8
  Switch Case/1 -> 1B/Action
  1B7/1(Out1) -> Index Vector/9
  1B5/1(Out1) -> Index Vector/7
  Index Vector/1 -> Generated Field/1

== system can8auto/SYNC PRODUCER/CAN NODE/PDO Frame Generator/Switch Case Action Subsystem ==
  In1 : Inport
  Action Port : ActionPort  ActionType=case
  Out1 : Outport
  wires:
  In1/1 -> Out1/1

== system can8auto/SYNC PRODUCER/CAN NODE/PDO Frame Generator/Switch Case Action Subsystem1 ==
  In1 : Inport
  Action Port : ActionPort  ActionType=case
  Out1 : Outport
  wires:
  In1/1 -> Out1/1

== system can8auto/SYNC PRODUCER/CAN NODE/PDO Frame Generator/Switch Case Action Subsystem2 ==
  In1 : Inport
  Action Port : ActionPort  ActionType=default
  Out1 : Outport
  wires:
  In1/1 -> Out1/1

== system can8auto/SYNC PRODUCER/CAN NODE/SDO Frame generator/BitStuffing ==
  In1 : Inport
  MATLAB Function : MATLAB Function  TreatAsAtomicUnit=on
  Out1 : Outport
  wires:
  In1/1 -> MATLAB Function/1(u)
  MATLAB Function/1(b) -> Out1/1

== system can8auto/SYNC PRODUCER/CAN NODE/SDO Frame generator/MUX ==
  Mode : Inport
  Read Client Data : Inport  Port=2
  Write Client Data : Inport  Port=3
  Read Server Data : Inport  Port=4
  Write Server Data : Inport  Port=5
  Complex to Real-Imag : ComplexToRealImag  Output=Real
  MATLAB Function : MATLAB Function  TreatAsAtomicUnit=on
  Vector Concatenate5 : Concatenate  NumInputs=4
  Data to Frame : Outport
  wires:
  Read Server Data/1 -> Vector Concatenate5/3
  Complex to Real-Imag/1 -> Data to Frame/1
  MATLAB Function/1(result) -> Complex to Real-Imag/1
  Read Client Data/1 -> Vector Concatenate5/1
  Vector Concatenate5/1 -> MATLAB Function/2(u1)
  Write Server Data/1 -> Vector Concatenate5/4
  Mode/1 -> MATLAB Function/1(index)
  Write Client Data/1 -> Vector Concatenate5/2

== system can8auto/SYNC PRODUCER/CAN NODE/SDO Frame generator/Subsystem ==
  Random Bits : Inport
  Length of Field : Inport  Port=2
  1B : Subsystem  TreatAsAtomicUnit=on
  1B1 : Subsystem  TreatAsAtomicUnit=on
  1B2 : Subsystem  TreatAsAtomicUnit=on
  1B3 : Subsystem  TreatAsAtomicUnit=on
  1B4 : Subsystem  TreatAsAtomicUnit=on
  1B5 : Subsystem  TreatAsAtomicUnit=on
  1B6 : Subsystem  TreatAsAtomicUnit=on
  1B7 : Subsystem  TreatAsAtomicUnit=on
  Demux : Demux  Outputs=8
  Index Vector : MultiPortSwitch  Inputs=8  AllowDiffInputSizes=on
  Switch Case : SwitchCase  CaseConditions={1,2,3,4,5,6,7}
  Generated Field : Outport
  wires:
  Switch Case/8 -> 1B7/Action
  1B/1(Out1) -> Index Vector/2
  Demux/3 -> 1B2/3(In3), 1B6/3(In3), 1B4/3(In3), 1B3/3(In3), 1B7/3(In3), 1B5/3(In3)
  Random Bits/1 -> Demux/1
  Switch Case/3 -> 1B2/Action
  Switch Case/6 -> 1B5/Action
  Demux/2 -> 1B2/2(In2), 1B3/2(In2), 1B4/2(In2), 1B5/2(In2), 1B7/2(In2), 1B6/2(In2), 1B1/2(In2)
  1B2/1(Out1) -> Index Vector/4
  Switch Case/5 -> 1B4/Action
  1B3/1(Out1) -> Index Vector/5
  Demux/1 -> 1B1/1(In1), 1B/1(In1), 1B2/1(In1), 1B3/1(In1), 1B4/1(In1), 1B5/1(In1), 1B6/1(In1), 1B7/1(In1)
  Switch Case/2 -> 1B1/Action
  Switch Case/7 -> 1B6/Action
  Demux/4 -> 1B6/4(In4), 1B3/4(In4), 1B7/4(In4), 1B4/4(In4), 1B5/4(In4)
  1B1/1(Out1) -> Index Vector/3
  1B4/1(Out1) -> Index Vector/6
  Demux/8 -> 1B7/8(In8)
  Demux/7 -> 1B6/7(In7), 1B7/7(In7)
  Length of Field/1 -> Switch Case/1, Index Vector/1
  Switch Case/4 -> 1B3/Action
  Demux/5 -> 1B4/5(In5), 1B7/5(In5), 1B6/5(In5), 1B5/5(In5)
  Demux/6 -> 1B5/6(In6), 1B6/6(In6), 1B7/6(In6)
  1B6/1(Out1) -> Index Vector/8
  Switch Case/1 -> 1B/Action
  1B7/1(Out1) -> Index Vector/9
  1B5/1(Out1) -> Index Vector/7
  Index Vector/1 -> Generated Field/1

== system can8auto/SYNC PRODUCER/CAN NODE/SDO Frame generator/Subsystem1 ==
  Random Bits : Inport
  Length of Field : Inport  Port=2
  1B : Subsystem  TreatAsAtomicUnit=on
  1B1 : Subsystem  TreatAsAtomicUnit=on
  1B2 : Subsystem  TreatAsAtomicUnit=on
  1B3 : Subsystem  TreatAsAtomicUnit=on
  1B4 : Subsystem  TreatAsAtomicUnit=on
  1B5 : Subsystem  TreatAsAtomicUnit=on
  1B6 : Subsystem  TreatAsAtomicUnit=on
  1B7 : Subsystem  TreatAsAtomicUnit=on
  Demux : Demux  Outputs=8
  Index Vector : MultiPortSwitch  Inputs=8  AllowDiffInputSizes=on
  Switch Case : SwitchCase  CaseConditions={1,2,3,4,5,6,7}
  Generated Field : Outport
  wires:
  Switch Case/8 -> 1B7/Action
  1B/1(Out1) -> Index Vector/2
  Demux/3 -> 1B2/3(In3), 1B6/3(In3), 1B4/3(In3), 1B3/3(In3), 1B7/3(In3), 1B5/3(In3)
  Random Bits/1 -> Demux/1
  Switch Case/3 -> 1B2/Action
  Switch Case/6 -> 1B5/Action
  Demux/2 -> 1B2/2(In2), 1B3/2(In2), 1B4/2(In2), 1B5/2(In2), 1B7/2(In2), 1B6/2(In2), 1B1/2(In2)
  1B2/1(Out1) -> Index Vector/4
  Switch Case/5 -> 1B4/Action
  1B3/1(Out1) -> Index Vector/5
  Demux/1 -> 1B1/1(In1), 1B/1(In1), 1B2/1(In1), 1B3/1(In1), 1B4/1(In1), 1B5/1(In1), 1B6/1(In1), 1B7/1(In1)
  Switch Case/2 -> 1B1/Action
  Switch Case/7 -> 1B6/Action
  Demux/4 -> 1B6/4(In4), 1B3/4(In4), 1B7/4(In4), 1B4/4(In4), 1B5/4(In4)
  1B1/1(Out1) -> Index Vector/3
  1B4/1(Out1) -> Index Vector/6
  Demux/8 -> 1B7/8(In8)
  Demux/7 -> 1B6/7(In7), 1B7/7(In7)
  Length of Field/1 -> Index Vector/1, Switch Case/1
  Switch Case/4 -> 1B3/Action
  Demux/5 -> 1B4/5(In5), 1B7/5(In5), 1B6/5(In5), 1B5/5(In5)
  Demux/6 -> 1B5/6(In6), 1B6/6(In6), 1B7/6(In6)
  1B6/1(Out1) -> Index Vector/8
  Switch Case/1 -> 1B/Action
  1B7/1(Out1) -> Index Vector/9
  1B5/1(Out1) -> Index Vector/7
  Index Vector/1 -> Generated Field/1

== system can8auto/SYNC PRODUCER/CAN NODE/SDO Frame generator/Subsystem2 ==
  Random Bits : Inport
  Length of Field : Inport  Port=2
  1B : Subsystem  TreatAsAtomicUnit=on
  1B1 : Subsystem  TreatAsAtomicUnit=on
  1B2 : Subsystem  TreatAsAtomicUnit=on
  1B3 : Subsystem  TreatAsAtomicUnit=on
  1B4 : Subsystem  TreatAsAtomicUnit=on
  1B5 : Subsystem  TreatAsAtomicUnit=on
  1B6 : Subsystem  TreatAsAtomicUnit=on
  1B7 : Subsystem  TreatAsAtomicUnit=on
  Demux : Demux  Outputs=8
  Index Vector : MultiPortSwitch  Inputs=8  AllowDiffInputSizes=on
  Switch Case : SwitchCase  CaseConditions={1,2,3,4,5,6,7}
  Generated Field : Outport
  wires:
  Switch Case/8 -> 1B7/Action
  1B/1(Out1) -> Index Vector/2
  Demux/3 -> 1B2/3(In3), 1B6/3(In3), 1B4/3(In3), 1B3/3(In3), 1B7/3(In3), 1B5/3(In3)
  Random Bits/1 -> Demux/1
  Switch Case/3 -> 1B2/Action
  Switch Case/6 -> 1B5/Action
  Demux/2 -> 1B2/2(In2), 1B3/2(In2), 1B4/2(In2), 1B5/2(In2), 1B7/2(In2), 1B6/2(In2), 1B1/2(In2)
  1B2/1(Out1) -> Index Vector/4
  Switch Case/5 -> 1B4/Action
  1B3/1(Out1) -> Index Vector/5
  Demux/1 -> 1B1/1(In1), 1B/1(In1), 1B2/1(In1), 1B3/1(In1), 1B4/1(In1), 1B5/1(In1), 1B6/1(In1), 1B7/1(In1)
  Switch Case/2 -> 1B1/Action
  Switch Case/7 -> 1B6/Action
  Demux/4 -> 1B6/4(In4), 1B3/4(In4), 1B7/4(In4), 1B4/4(In4), 1B5/4(In4)
  1B1/1(Out1) -> Index Vector/3
  1B4/1(Out1) -> Index Vector/6
  Demux/8 -> 1B7/8(In8)
  Demux/7 -> 1B6/7(In7), 1B7/7(In7)
  Length of Field/1 -> Switch Case/1, Index Vector/1
  Switch Case/4 -> 1B3/Action
  Demux/5 -> 1B4/5(In5), 1B7/5(In5), 1B6/5(In5), 1B5/5(In5)
  Demux/6 -> 1B5/6(In6), 1B6/6(In6), 1B7/6(In6)
  1B6/1(Out1) -> Index Vector/8
  Switch Case/1 -> 1B/Action
  1B7/1(Out1) -> Index Vector/9
  1B5/1(Out1) -> Index Vector/7
  Index Vector/1 -> Generated Field/1

== system can8auto/SYNC PRODUCER/CAN NODE/SDO Frame generator/Subsystem3 ==
  Random Bits : Inport
  Length of Field : Inport  Port=2
  1B : Subsystem  TreatAsAtomicUnit=on
  1B1 : Subsystem  TreatAsAtomicUnit=on
  1B2 : Subsystem  TreatAsAtomicUnit=on
  1B3 : Subsystem  TreatAsAtomicUnit=on
  1B4 : Subsystem  TreatAsAtomicUnit=on
  1B5 : Subsystem  TreatAsAtomicUnit=on
  1B6 : Subsystem  TreatAsAtomicUnit=on
  1B7 : Subsystem  TreatAsAtomicUnit=on
  Demux : Demux  Outputs=8
  Index Vector : MultiPortSwitch  Inputs=8  AllowDiffInputSizes=on
  Switch Case : SwitchCase  CaseConditions={1,2,3,4,5,6,7}
  Generated Field : Outport
  wires:
  Switch Case/8 -> 1B7/Action
  1B/1(Out1) -> Index Vector/2
  Demux/3 -> 1B2/3(In3), 1B6/3(In3), 1B4/3(In3), 1B3/3(In3), 1B7/3(In3), 1B5/3(In3)
  Random Bits/1 -> Demux/1
  Switch Case/3 -> 1B2/Action
  Switch Case/6 -> 1B5/Action
  Demux/2 -> 1B2/2(In2), 1B3/2(In2), 1B4/2(In2), 1B5/2(In2), 1B7/2(In2), 1B6/2(In2), 1B1/2(In2)
  1B2/1(Out1) -> Index Vector/4
  Switch Case/5 -> 1B4/Action
  1B3/1(Out1) -> Index Vector/5
  Demux/1 -> 1B1/1(In1), 1B/1(In1), 1B2/1(In1), 1B3/1(In1), 1B4/1(In1), 1B5/1(In1), 1B6/1(In1), 1B7/1(In1)
  Switch Case/2 -> 1B1/Action
  Switch Case/7 -> 1B6/Action
  Demux/4 -> 1B6/4(In4), 1B3/4(In4), 1B7/4(In4), 1B4/4(In4), 1B5/4(In4)
  1B1/1(Out1) -> Index Vector/3
  1B4/1(Out1) -> Index Vector/6
  Demux/8 -> 1B7/8(In8)
  Demux/7 -> 1B6/7(In7), 1B7/7(In7)
  Length of Field/1 -> Switch Case/1, Index Vector/1
  Switch Case/4 -> 1B3/Action
  Demux/5 -> 1B4/5(In5), 1B7/5(In5), 1B6/5(In5), 1B5/5(In5)
  Demux/6 -> 1B5/6(In6), 1B6/6(In6), 1B7/6(In6)
  1B6/1(Out1) -> Index Vector/8
  Switch Case/1 -> 1B/Action
  1B7/1(Out1) -> Index Vector/9
  1B5/1(Out1) -> Index Vector/7
  Index Vector/1 -> Generated Field/1

== system can8auto/SYNC PRODUCER/CAN NODE/SYNC Frame Generator/BitStuffing ==
  In1 : Inport
  MATLAB Function : MATLAB Function  TreatAsAtomicUnit=on
  Out1 : Outport
  wires:
  In1/1 -> MATLAB Function/1(u)
  MATLAB Function/1(b) -> Out1/1

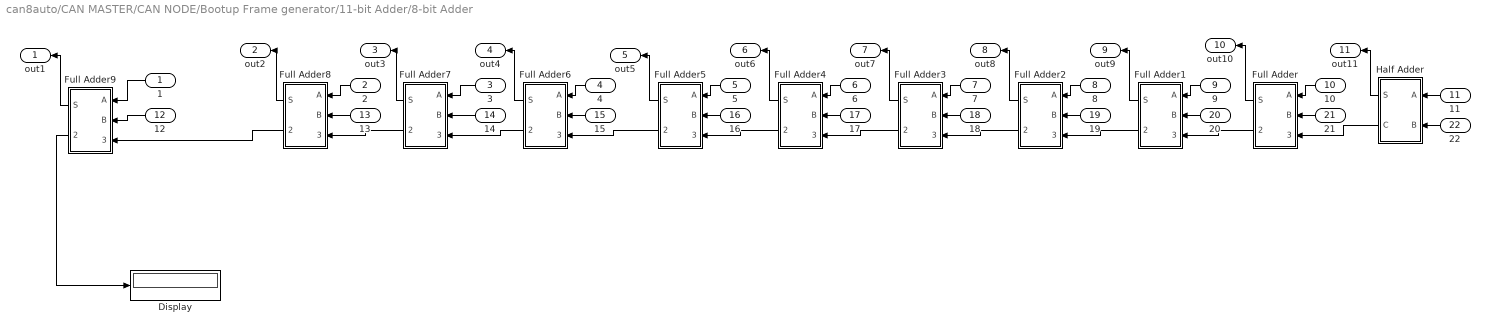
== system can8auto/CAN MASTER/CAN NODE/Bootup Frame generator/11-bit Adder/8-bit Adder ==
  1 : Inport
  2 : Inport  Port=2
  3 : Inport  Port=3
  4 : Inport  Port=4
  5 : Inport  Port=5
  6 : Inport  Port=6
  7 : Inport  Port=7
  8 : Inport  Port=8
  9 : Inport  Port=9
  10 : Inport  Port=10
  11 : Inport  Port=11
  12 : Inport  Port=12
  13 : Inport  Port=13
  14 : Inport  Port=14
  15 : Inport  Port=15
  16 : Inport  Port=16
  17 : Inport  Port=17
  18 : Inport  Port=18
  19 : Inport  Port=19
  20 : Inport  Port=20
  21 : Inport  Port=21
  22 : Inport  Port=22
  Display : Display
  Full Adder : Subsystem
  Full Adder1 : Subsystem
  Full Adder2 : Subsystem
  Full Adder3 : Subsystem
  Full Adder4 : Subsystem
  Full Adder5 : Subsystem
  Full Adder6 : Subsystem
  Full Adder7 : Subsystem
  Full Adder8 : Subsystem
  Full Adder9 : Subsystem
  Half Adder : Subsystem
  out1 : Outport
  out2 : Outport  Port=2
  out3 : Outport  Port=3
  out4 : Outport  Port=4
  out5 : Outport  Port=5
  out6 : Outport  Port=6
  out7 : Outport  Port=7
  out8 : Outport  Port=8
  out9 : Outport  Port=9
  out10 : Outport  Port=10
  out11 : Outport  Port=11
  wires:
  Full Adder9/2(Cout) -> Display/1
  1/1 -> Full Adder9/1(A)
  12/1 -> Full Adder9/2(B)
  13/1 -> Full Adder8/2(B)
  2/1 -> Full Adder8/1(A)
  14/1 -> Full Adder7/2(B)
  3/1 -> Full Adder7/1(A)
  Full Adder8/2(Cout) -> Full Adder9/3(Cin)
  Full Adder7/2(Cout) -> Full Adder8/3(Cin)
  Full Adder9/1(S) -> out1/1
  Full Adder8/1(S) -> out2/1
  Full Adder7/1(S) -> out3/1
  Full Adder6/2(Cout) -> Full Adder7/3(Cin)
  Half Adder/1(S) -> out11/1
  Full Adder4/1(S) -> out6/1
  Full Adder2/1(S) -> out8/1
  5/1 -> Full Adder5/1(A)
  22/1 -> Half Adder/2(B)
  Full Adder3/2(Cout) -> Full Adder4/3(Cin)
  Half Adder/2(C) -> Full Adder/3(Cin)
  Full Adder4/2(Cout) -> Full Adder5/3(Cin)
  Full Adder1/2(Cout) -> Full Adder2/3(Cin)
  Full Adder3/1(S) -> out7/1
  7/1 -> Full Adder3/1(A)
  Full Adder5/1(S) -> out5/1
  15/1 -> Full Adder6/2(B)
  19/1 -> Full Adder2/2(B)
  17/1 -> Full Adder4/2(B)
  16/1 -> Full Adder5/2(B)
  Full Adder/2(Cout) -> Full Adder1/3(Cin)
  20/1 -> Full Adder1/2(B)
  Full Adder1/1(S) -> out9/1
  6/1 -> Full Adder4/1(A)
  10/1 -> Full Adder/1(A)
  18/1 -> Full Adder3/2(B)
  4/1 -> Full Adder6/1(A)
  Full Adder6/1(S) -> out4/1
  21/1 -> Full Adder/2(B)
  Full Adder5/2(Cout) -> Full Adder6/3(Cin)
  Full Adder2/2(Cout) -> Full Adder3/3(Cin)
  11/1 -> Half Adder/1(A)
  9/1 -> Full Adder1/1(A)
  Full Adder/1(S) -> out10/1
  8/1 -> Full Adder2/1(A)

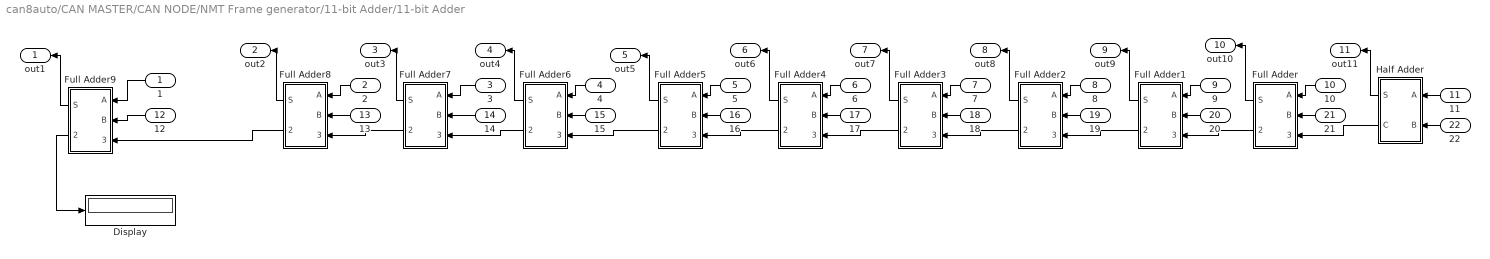
== system can8auto/CAN MASTER/CAN NODE/NMT Frame generator/11-bit Adder/11-bit Adder ==
  1 : Inport
  2 : Inport  Port=2
  3 : Inport  Port=3
  4 : Inport  Port=4
  5 : Inport  Port=5
  6 : Inport  Port=6
  7 : Inport  Port=7
  8 : Inport  Port=8
  9 : Inport  Port=9
  10 : Inport  Port=10
  11 : Inport  Port=11
  12 : Inport  Port=12
  13 : Inport  Port=13
  14 : Inport  Port=14
  15 : Inport  Port=15
  16 : Inport  Port=16
  17 : Inport  Port=17
  18 : Inport  Port=18
  19 : Inport  Port=19
  20 : Inport  Port=20
  21 : Inport  Port=21
  22 : Inport  Port=22
  Display : Display
  Full Adder : Subsystem
  Full Adder1 : Subsystem
  Full Adder2 : Subsystem
  Full Adder3 : Subsystem
  Full Adder4 : Subsystem
  Full Adder5 : Subsystem
  Full Adder6 : Subsystem
  Full Adder7 : Subsystem
  Full Adder8 : Subsystem
  Full Adder9 : Subsystem
  Half Adder : Subsystem
  out1 : Outport
  out2 : Outport  Port=2
  out3 : Outport  Port=3
  out4 : Outport  Port=4
  out5 : Outport  Port=5
  out6 : Outport  Port=6
  out7 : Outport  Port=7
  out8 : Outport  Port=8
  out9 : Outport  Port=9
  out10 : Outport  Port=10
  out11 : Outport  Port=11
  wires:
  Full Adder9/2(Cout) -> Display/1
  1/1 -> Full Adder9/1(A)
  12/1 -> Full Adder9/2(B)
  13/1 -> Full Adder8/2(B)
  2/1 -> Full Adder8/1(A)
  14/1 -> Full Adder7/2(B)
  3/1 -> Full Adder7/1(A)
  Full Adder8/2(Cout) -> Full Adder9/3(Cin)
  Full Adder7/2(Cout) -> Full Adder8/3(Cin)
  Full Adder9/1(S) -> out1/1
  Full Adder8/1(S) -> out2/1
  Full Adder7/1(S) -> out3/1
  Full Adder6/2(Cout) -> Full Adder7/3(Cin)
  Half Adder/1(S) -> out11/1
  Full Adder4/1(S) -> out6/1
  Full Adder2/1(S) -> out8/1
  5/1 -> Full Adder5/1(A)
  22/1 -> Half Adder/2(B)
  Full Adder3/2(Cout) -> Full Adder4/3(Cin)
  Half Adder/2(C) -> Full Adder/3(Cin)
  Full Adder4/2(Cout) -> Full Adder5/3(Cin)
  Full Adder1/2(Cout) -> Full Adder2/3(Cin)
  Full Adder3/1(S) -> out7/1
  7/1 -> Full Adder3/1(A)
  Full Adder5/1(S) -> out5/1
  15/1 -> Full Adder6/2(B)
  19/1 -> Full Adder2/2(B)
  17/1 -> Full Adder4/2(B)
  16/1 -> Full Adder5/2(B)
  Full Adder/2(Cout) -> Full Adder1/3(Cin)
  20/1 -> Full Adder1/2(B)
  Full Adder1/1(S) -> out9/1
  6/1 -> Full Adder4/1(A)
  10/1 -> Full Adder/1(A)
  18/1 -> Full Adder3/2(B)
  4/1 -> Full Adder6/1(A)
  Full Adder6/1(S) -> out4/1
  21/1 -> Full Adder/2(B)
  Full Adder5/2(Cout) -> Full Adder6/3(Cin)
  Full Adder2/2(Cout) -> Full Adder3/3(Cin)
  11/1 -> Half Adder/1(A)
  9/1 -> Full Adder1/1(A)
  Full Adder/1(S) -> out10/1
  8/1 -> Full Adder2/1(A)

== system can8auto/CAN MASTER/CAN NODE/PDO Frame Generator/Subsystem/1B ==
  In1 : Inport
  Action Port : ActionPort  ActionType=case
  Out1 : Outport
  wires:
  In1/1 -> Out1/1

== system can8auto/CAN MASTER/CAN NODE/PDO Frame Generator/Subsystem/1B1 ==
  In1 : Inport
  In2 : Inport  Port=2
  Action Port : ActionPort  ActionType=case
  Mux : Mux  Inputs=2
  Out1 : Outport
  wires:
  Mux/1 -> Out1/1
  In2/1 -> Mux/2
  In1/1 -> Mux/1

== system can8auto/CAN MASTER/CAN NODE/PDO Frame Generator/Subsystem/1B2 ==
  In1 : Inport
  In2 : Inport  Port=2
  In3 : Inport  Port=3
  Action Port : ActionPort  ActionType=case
  Mux : Mux  Inputs=3
  Out1 : Outport
  wires:
  In3/1 -> Mux/3
  Mux/1 -> Out1/1
  In2/1 -> Mux/2
  In1/1 -> Mux/1

== system can8auto/CAN MASTER/CAN NODE/PDO Frame Generator/Subsystem/1B3 ==
  In1 : Inport
  In2 : Inport  Port=2
  In3 : Inport  Port=3
  In4 : Inport  Port=4
  Action Port : ActionPort  ActionType=case
  Mux : Mux
  Out1 : Outport
  wires:
  In4/1 -> Mux/4
  In3/1 -> Mux/3
  Mux/1 -> Out1/1
  In2/1 -> Mux/2
  In1/1 -> Mux/1

== system can8auto/CAN MASTER/CAN NODE/PDO Frame Generator/Subsystem/1B4 ==
  In1 : Inport
  In2 : Inport  Port=2
  In3 : Inport  Port=3
  In4 : Inport  Port=4
  In5 : Inport  Port=5
  Action Port : ActionPort  ActionType=case
  Mux : Mux  Inputs=5
  Out1 : Outport
  wires:
  In5/1 -> Mux/5
  In4/1 -> Mux/4
  In3/1 -> Mux/3
  Mux/1 -> Out1/1
  In2/1 -> Mux/2
  In1/1 -> Mux/1

== system can8auto/CAN MASTER/CAN NODE/PDO Frame Generator/Subsystem/1B5 ==
  In1 : Inport
  In2 : Inport  Port=2
  In3 : Inport  Port=3
  In4 : Inport  Port=4
  In5 : Inport  Port=5
  In6 : Inport  Port=6
  Action Port : ActionPort  ActionType=case
  Mux : Mux  Inputs=6
  Out1 : Outport
  wires:
  In6/1 -> Mux/6
  In5/1 -> Mux/5
  In4/1 -> Mux/4
  In3/1 -> Mux/3
  Mux/1 -> Out1/1
  In2/1 -> Mux/2
  In1/1 -> Mux/1

== system can8auto/CAN MASTER/CAN NODE/PDO Frame Generator/Subsystem/1B6 ==
  In1 : Inport
  In2 : Inport  Port=2
  In3 : Inport  Port=3
  In4 : Inport  Port=4
  In5 : Inport  Port=5
  In6 : Inport  Port=6
  In7 : Inport  Port=7
  Action Port : ActionPort  ActionType=case
  Mux : Mux  Inputs=7
  Out1 : Outport
  wires:
  In7/1 -> Mux/7
  In6/1 -> Mux/6
  In5/1 -> Mux/5
  In4/1 -> Mux/4
  In3/1 -> Mux/3
  Mux/1 -> Out1/1
  In2/1 -> Mux/2
  In1/1 -> Mux/1

== system can8auto/CAN MASTER/CAN NODE/PDO Frame Generator/Subsystem/1B7 ==
  In1 : Inport
  In2 : Inport  Port=2
  In3 : Inport  Port=3
  In4 : Inport  Port=4
  In5 : Inport  Port=5
  In6 : Inport  Port=6
  In7 : Inport  Port=7
  In8 : Inport  Port=8
  Action Port : ActionPort  ActionType=default
  Mux : Mux  Inputs=8
  Out1 : Outport
  wires:
  In8/1 -> Mux/8
  In7/1 -> Mux/7
  In6/1 -> Mux/6
  In5/1 -> Mux/5
  In4/1 -> Mux/4
  In3/1 -> Mux/3
  Mux/1 -> Out1/1
  In2/1 -> Mux/2
  In1/1 -> Mux/1

== system can8auto/CAN MASTER/CAN NODE/SDO Frame generator/Subsystem/1B ==
  In1 : Inport
  Action Port : ActionPort  ActionType=case
  Out1 : Outport
  wires:
  In1/1 -> Out1/1

== system can8auto/CAN MASTER/CAN NODE/SDO Frame generator/Subsystem/1B1 ==
  In1 : Inport
  In2 : Inport  Port=2
  Action Port : ActionPort  ActionType=case
  Mux : Mux  Inputs=2
  Out1 : Outport
  wires:
  Mux/1 -> Out1/1
  In2/1 -> Mux/2
  In1/1 -> Mux/1

== system can8auto/CAN MASTER/CAN NODE/SDO Frame generator/Subsystem/1B2 ==
  In1 : Inport
  In2 : Inport  Port=2
  In3 : Inport  Port=3
  Action Port : ActionPort  ActionType=case
  Mux : Mux  Inputs=3
  Out1 : Outport
  wires:
  In3/1 -> Mux/3
  Mux/1 -> Out1/1
  In2/1 -> Mux/2
  In1/1 -> Mux/1
